simulink model "exampleModel_bus_axi_w_4ptavg"  (R2017b)
settings: Solver=VariableStepAuto  StartTime=0.0  StopTime=10e-5  RelTol=1e-3
PreLoadFcn:
  | setup
values from neighbouring files (symbols this model uses):
  axiClk = 156.25e6    (= 156250000)    [setup.m]    (also in setup_exampleModel_bus_axi_simulink.m; setup_exampleModel_bus_axi_simulink_lcls2.m; setup_lcls2_pcav.m; sysgen_signal.m)
  cav1p1_addr = 204    [setup_exampleModel_bus_axi_simulink.m]    (also in setup_exampleModel_bus_axi_simulink_lcls2.m; setup_lcls2_pcav.m; sysgen_signal.m)
  cav1p2_addr = cav1p1_addr * 2    (= 408)    [setup_exampleModel_bus_axi_simulink.m]    (also in setup_exampleModel_bus_axi_simulink_lcls2.m; setup_lcls2_pcav.m; sysgen_signal.m)
  cav2p1_addr = cav1p1_addr * 3    (= 612)    [setup_exampleModel_bus_axi_simulink.m]    (also in setup_exampleModel_bus_axi_simulink_lcls2.m; setup_lcls2_pcav.m; sysgen_signal.m)
  cav2p2_addr = cav1p1_addr * 4    (= 816)    [setup_exampleModel_bus_axi_simulink.m]    (also in setup_exampleModel_bus_axi_simulink_lcls2.m; setup_lcls2_pcav.m; sysgen_signal.m)
  Fadc = Fs/interleavedChannels    (= 29750000)    [setup.m]    (also in setup_exampleModel_bus_axi_simulink.m = 357000000; setup_exampleModel_bus_axi_simulink_lcls2.m = 351000000; setup_lcls2_pcav.m = 357000000; sysgen_signal.m = 357000000)
  fir_lpf = fir1(15, w_lpf)    [setup_exampleModel_bus_axi_simulink.m]    (also in setup_exampleModel_bus_axi_simulink_lcls2.m; setup_lcls2_pcav.m)
  Fproc = 204e6    (= 204000000)    [setup_exampleModel_bus_axi_simulink.m]    (also in setup_exampleModel_bus_axi_simulink_lcls2.m = 200571400; setup_lcls2_pcav.m; sysgen_signal.m)
  Fsig = Fproc/12    (= 17000000)    [setup_exampleModel_bus_axi_simulink.m]    (also in setup_exampleModel_bus_axi_simulink_lcls2.m = 16714283.3333; setup_lcls2_pcav.m)
  Tadc = 1/fadc    (= 2.80112044818e-09)    [cavity_signal.m]    (also in setup_exampleModel_bus_axi_simulink.m; setup_exampleModel_bus_axi_simulink_lcls2.m = 2.849002849e-09; setup_lcls2_pcav.m; setup_pcav_simulink.m)
undefined symbols (not defined in the file or in its folder): AXI4, Lite
libraries: xbsIndex_r4 x2870, llrf_lib x10, simulink x3
(part 7 of 15)

== system exampleModel_bus_axi_w_4ptavg/example/dsp/Cav1/Subsystem ==
  In1 : Inport
  In2 : Inport  Port=2
  In3 : Inport  Port=3
  In4 : Inport  Port=4
  AddSub1 : xbsIndex_r4/AddSub  mode=Addition  use_carryin=off  use_carryout=off  en=off  latency=1  precision=User Defined  arith_type=Unsigned  n_bits=16  bin_pt=0  quantization=Truncate  overflow=Wrap  use_behavioral_HDL=off  hw_selection=Fabric  pipelined=off  dbl_ovrd=off  block_type=addsub
  AddSub2 : xbsIndex_r4/AddSub  mode=Addition  use_carryin=off  use_carryout=off  en=off  latency=1  precision=User Defined  arith_type=Unsigned  n_bits=16  bin_pt=0  quantization=Truncate  overflow=Wrap  use_behavioral_HDL=off  hw_selection=Fabric  pipelined=off  dbl_ovrd=off  block_type=addsub
  CORDIC 6.0 1 : xbsIndex_r4/CORDIC 6.0   functional_selection=Translate  architectural_configuration=Parallel  pipelining_mode=Maximum  data_format=SignedFraction  phase_format=Scaled_Radians  input_width=33  output_width=33  round_mode=Truncate  iterations=0  precision=0  compensation_scaling=No_Scale_Compensation  coarse_rotation=on  aclken=off  aresetn=off  out_tready=off  cartesian_has_tuser=off  cartesian_has_tlast=off  cartesian_tuser_width=1  phase_has_tuser=off  phase_has_tlast=off  phase_tuser_width=1  out_tlast_behv=Null  flow_control=NonBlocking  optimize_goal=Resources  trim_axipin_name=on  simulation_type=hybrid_sim  simulation_model=sysgen:cordic_v6_0  data_path_portlist={'s_axis_cartesian_tdata_imag', 's_axis_cartesian_tdata_real', 's_axis_phase_tdata_phase', 'm_axis_dout_tdata_imag', 'm_axis_dout_tdata_real', 'm_axis_dout_tdata_phase','m_axis_dout_tdata'}  ip_name=CORDIC  ip_version=6.0  dsptool_ready=true  ipcore_usecache=true  ipcore_useipmodelcache=true  wrapper_available=true  port_translation_map={ 'aclken' => 'en', 'aresetn' => 'rst' }  block_type=cordic_v6_0
      settings: infoedit=CORDIC 6.0
  Clock Enable Probe3 : xbsIndex_r4/Clock Enable Probe  inherit_constraints=on  block_type=ceprobe
      settings: infoedit="Clock enable extractor.  Produces a Boolean output that mirrors the hardware clock enable associated with the input sample rate.<br><br>Hardware notes: in hardware this block costs nothing."
  Constant13 : xbsIndex_r4/Constant  const=0  gui_display_data_type=Boolean  arith_type=Boolean  n_bits=16  bin_pt=14  preci_type=Single  exp_width=8  frac_width=24  explicit_period=off  period=1  equ=P=C  opselect=C  inp2=PCIN>>17  opr=+  inp1=P  carry=CIN  dbl_ovrd=off  block_type=constant
  Constant15 : xbsIndex_r4/Constant  const=0  gui_display_data_type=Fixed-point  arith_type=Signed (2's comp)  n_bits=33  bin_pt=31  preci_type=Single  exp_width=8  frac_width=24  explicit_period=off  period=1  equ=P=C  opselect=C  inp2=PCIN>>17  opr=+  inp1=P  carry=CIN  dbl_ovrd=off  block_type=constant
  Constant3 : xbsIndex_r4/Constant  const=1.0  gui_display_data_type=Boolean  arith_type=Boolean  n_bits=16  bin_pt=14  preci_type=Single  exp_width=8  frac_width=24  explicit_period=off  period=1  equ=P=C  opselect=C  inp2=PCIN>>17  opr=+  inp1=P  carry=CIN  dbl_ovrd=off  block_type=constant
  Constant4 : xbsIndex_r4/Constant  const=0  gui_display_data_type=Boolean  arith_type=Boolean  n_bits=16  bin_pt=14  preci_type=Single  exp_width=8  frac_width=24  explicit_period=off  period=1  equ=P=C  opselect=C  inp2=PCIN>>17  opr=+  inp1=P  carry=CIN  dbl_ovrd=off  block_type=constant
  Constant5 : xbsIndex_r4/Constant  const=0  gui_display_data_type=Fixed-point  arith_type=Signed (2's comp)  n_bits=33  bin_pt=31  preci_type=Single  exp_width=8  frac_width=24  explicit_period=off  period=1  equ=P=C  opselect=C  inp2=PCIN>>17  opr=+  inp1=P  carry=CIN  dbl_ovrd=off  block_type=constant
  Constant6 : xbsIndex_r4/Constant  const=1.0  gui_display_data_type=Boolean  arith_type=Boolean  n_bits=16  bin_pt=14  preci_type=Single  exp_width=8  frac_width=24  explicit_period=off  period=1  equ=P=C  opselect=C  inp2=PCIN>>17  opr=+  inp1=P  carry=CIN  dbl_ovrd=off  block_type=constant
  Down Sample8 : xbsIndex_r4/Down Sample  sample_ratio=12  sample_phase="Last Value of Frame  (most efficient)"  en=off  rst=off  latency=1  dbl_ovrd=off  block_type=dsamp
  Dual Port RAM : xbsIndex_r4/Dual Port RAM  depth=2^16  initVector=zeros(1,2^8)  distributed_mem=Block RAM  init_a=0  init_b=0  rst_a=off  rst_b=off  en_a=off  en_b=off  latency=1  write_mode_A=Read Before Write  write_mode_B=Read Before Write  optimize=Area  dbl_ovrd=off  block_type=dpram
  Dual Port RAM1 : xbsIndex_r4/Dual Port RAM  depth=2^16  initVector=zeros(1,2^8)  distributed_mem=Block RAM  init_a=0  init_b=0  rst_a=off  rst_b=off  en_a=off  en_b=off  latency=1  write_mode_A=Read Before Write  write_mode_B=Read Before Write  optimize=Area  dbl_ovrd=off  block_type=dpram
  Gateway Out{7..11,20,22..24} (9 alike) : xbsIndex_r4/Gateway Out  inherit_from_input=off  hdl_port=off  rows=1  columns=1  UseAsDAC=off  DACChannel='1'  interface=None  automatic_assignment=on  address_offset=hex2dec('00')  intf_name=''  intf_description=''  timing_constraint=None  locs_specified=off  LOCs={}  io_standard={}  block_type=gatewayout
  Gateway Out{12..13,15,21,29} (5 alike) : xbsIndex_r4/Gateway Out  inherit_from_input=off  hdl_port=on  rows=1  columns=1  UseAsDAC=off  DACChannel='1'  interface=None  automatic_assignment=on  address_offset=hex2dec('00')  intf_name=''  intf_description=''  timing_constraint=None  locs_specified=off  LOCs={}  io_standard={}  block_type=gatewayout
  Mult1 : xbsIndex_r4/Mult  precision=User Defined  arith_type="Signed  (2's comp)"  n_bits=33  bin_pt=31  quantization=Truncate  overflow=Wrap  en=off  latency=3  use_behavioral_HDL=off  opt=Speed  use_embedded=on  optimum_pipeline=off  pipeline=on  dbl_ovrd=off  use_rpm=on  placement_style=Triangular  block_type=mult
  Mult3 : xbsIndex_r4/Mult  precision=User Defined  arith_type="Signed  (2's comp)"  n_bits=33  bin_pt=31  quantization=Truncate  overflow=Saturate  en=off  latency=3  use_behavioral_HDL=off  opt=Speed  use_embedded=on  optimum_pipeline=off  pipeline=on  dbl_ovrd=off  use_rpm=on  placement_style=Triangular  block_type=mult
  Scope10 : Scope  NumInputPorts=2
  Scope3 : Scope  NumInputPorts=3
  Scope6 : Scope  NumInputPorts=3
  Scope7 : Scope  NumInputPorts=4
  Scope8 : Scope  NumInputPorts=4
  Scope9 : Scope  NumInputPorts=2
  four_point_avg : Subsystem
  freq_err : Subsystem
  Out1 : Outport
  tag scope: Cav1_NCO_fb=global, delayed_test_img=global, delayed_test_real=global
  wires:
  In4/1 -> Scope7/4
  In3/1 -> Scope8/4
  In1/1 -> Scope3/3
  freq_err/1(NCO_err) -> [Cav1_NCO_fb]
  Gateway Out15/1 -> Scope7/2
  Dual Port RAM1/2 -> Gateway Out24/1, [delayed_test_real]
  Gateway Out24/1 -> Scope10/2
  [c1p2_pt_cntr] -> AddSub1/2, Dual Port RAM/4
  Constant15/1 -> Dual Port RAM/5
  Dual Port RAM/1 -> Gateway Out20/1
  [c1p2_pt_cntr] -> Dual Port RAM1/4, AddSub2/2
  AddSub2/1 -> Dual Port RAM1/1
  Gateway Out13/1 -> Scope8/3
  Constant13/1 -> Dual Port RAM/6
  Constant6/1 -> Dual Port RAM1/3
  In2/1 -> Scope7/3
  [c1p2_window_func] -> Mult3/2
  [test_img] -> Dual Port RAM/2
  Gateway Out22/1 -> Scope9/2
  AddSub1/1 -> Dual Port RAM/1
  Dual Port RAM1/1 -> Gateway Out23/1
  Constant5/1 -> Dual Port RAM1/5
  Gateway Out20/1 -> Scope9/1
  Constant3/1 -> Dual Port RAM/3
  CORDIC 6.0 1/3 -> Gateway Out9/1, Gateway Out7/1, four_point_avg/1(In1)
  CORDIC 6.0 1/1 -> Out1/1
  Gateway Out9/1 -> Scope6/1
  Clock Enable Probe3/1 -> Down Sample8/1
  Gateway Out23/1 -> Scope10/1
  [c1p2_delay_match] -> AddSub2/1
  Gateway Out11/1 -> Scope6/3
  Gateway Out21/1 -> Scope7/1
  Mult1/1 -> Gateway Out15/1, CORDIC 6.0 1/3
  Mult3/1 -> Gateway Out21/1, Clock Enable Probe3/1, CORDIC 6.0 1/2
  [c1p2_pt_cntr] -> Gateway Out11/1
  [delayed_test_img] -> Gateway Out29/1, Mult3/1
  Gateway Out12/1 -> Scope8/2
  Down Sample8/1 -> CORDIC 6.0 1/1
  [flo_c1p2_window] -> freq_err/2(window)
  [test_real] -> Dual Port RAM1/2
  Constant4/1 -> Dual Port RAM1/6
  [c1p2_window_func] -> Gateway Out13/1, Mult1/2
  Dual Port RAM/2 -> [delayed_test_img], Gateway Out22/1
  Gateway Out8/1 -> Scope3/2
  [dsp_cav1_reset] -> freq_err/3(reset)
  [delayed_test_real] -> Gateway Out12/1, Mult1/1
  CORDIC 6.0 1/2 -> Gateway Out10/1, freq_err/1(raw_phase)
  four_point_avg/1(Out1) -> Gateway Out8/1
  Gateway Out7/1 -> Scope3/1
  Gateway Out10/1 -> Scope6/2
  Gateway Out29/1 -> Scope8/1
  [c1p2_delay_match] -> AddSub1/1

== system exampleModel_bus_axi_w_4ptavg/example/dsp/Cav1/Subsystem1 ==
  IQ_stream_in : Inport
  IQ_chan_sel : Inport  Port=2
  Bus Creator5 : BusCreator  Inputs=3
  Bus Selector : BusSelector  OutputSignals=ddcI,ddcQ,sync
  Bus Selector3 : BusSelector  OutputSignals=ddcI,ddcQ,ddcSync,ddcChannel
  Channel Select3 : llrf_lib/Sysgen/Single Rate/Channel Select  SystemSampleTime=-1
      settings: SourceProductName=LLRF Library
  ddcI : Outport
  ddcQ : Outport  Port=2
  sync : Outport  Port=3
  wires:
  IQ_stream_in/1 -> Bus Selector3/1
  IQ_chan_sel/1 -> Channel Select3/5
  Channel Select3/3 -> Bus Creator5/3  "sync"
  Bus Selector3/2 -> Channel Select3/2  "<ddcQ>"
  Channel Select3/1 -> Bus Creator5/1  "ddcI"
  Channel Select3/2 -> Bus Creator5/2  "ddcQ"
  Bus Selector3/1 -> Channel Select3/1  "<ddcI>"
  Bus Selector3/4 -> Channel Select3/4  "<ddcChannel>"
  Bus Selector3/3 -> Channel Select3/3  "<ddcSync>"
  Bus Creator5/1 -> Bus Selector/1
  Bus Selector/1 -> ddcI/1  "<ddcI>"
  Bus Selector/2 -> ddcQ/1  "<ddcQ>"
  Bus Selector/3 -> sync/1  "<sync>"

== system exampleModel_bus_axi_w_4ptavg/example/dsp/Cav1/Subsystem10 ==
  d : Inport
  reset : Inport  Port=2
  cntr : Inport  Port=3
  threshold : Inport  Port=4
  Register11 : xbsIndex_r4/Register  init=0  rst=on  en=on  dbl_ovrd=off  block_type=register
  Relational4 : xbsIndex_r4/Relational  mode=a>b  op_type=Bool  en=off  latency=1  dbl_ovrd=off  block_type=relational
  posedge_pulse : Subsystem
  q : Outport
  wires:
  threshold/1 -> Relational4/2
  reset/1 -> Register11/2
  Relational4/1 -> posedge_pulse/1(In1)
  posedge_pulse/1(Out1) -> Register11/3
  Register11/1 -> q/1
  cntr/1 -> Relational4/1
  d/1 -> Register11/1

== system exampleModel_bus_axi_w_4ptavg/example/dsp/Cav1/Subsystem11 ==
  d : Inport
  reset : Inport  Port=2
  cntr : Inport  Port=3
  threshold : Inport  Port=4
  Register11 : xbsIndex_r4/Register  init=0  rst=on  en=on  dbl_ovrd=off  block_type=register
  Relational4 : xbsIndex_r4/Relational  mode=a>b  op_type=Bool  en=off  latency=1  dbl_ovrd=off  block_type=relational
  posedge_pulse : Subsystem
  q : Outport
  wires:
  d/1 -> Register11/1
  cntr/1 -> Relational4/1
  Register11/1 -> q/1
  posedge_pulse/1(Out1) -> Register11/3
  Relational4/1 -> posedge_pulse/1(In1)
  reset/1 -> Register11/2
  threshold/1 -> Relational4/2

== system exampleModel_bus_axi_w_4ptavg/example/dsp/Cav1/Subsystem12 ==
  d : Inport
  reset : Inport  Port=2
  cntr : Inport  Port=3
  threshold : Inport  Port=4
  Register11 : xbsIndex_r4/Register  init=0  rst=on  en=on  dbl_ovrd=off  block_type=register
  Relational4 : xbsIndex_r4/Relational  mode=a>b  op_type=Bool  en=off  latency=1  dbl_ovrd=off  block_type=relational
  posedge_pulse : Subsystem
  q : Outport
  wires:
  threshold/1 -> Relational4/2
  reset/1 -> Register11/2
  Relational4/1 -> posedge_pulse/1(In1)
  posedge_pulse/1(Out1) -> Register11/3
  Register11/1 -> q/1
  cntr/1 -> Relational4/1
  d/1 -> Register11/1

== system exampleModel_bus_axi_w_4ptavg/example/dsp/Cav1/Subsystem13 ==
  d : Inport
  reset : Inport  Port=2
  cntr : Inport  Port=3
  threshold : Inport  Port=4
  Register11 : xbsIndex_r4/Register  init=0  rst=on  en=on  dbl_ovrd=off  block_type=register
  Relational4 : xbsIndex_r4/Relational  mode=a>b  op_type=Bool  en=off  latency=1  dbl_ovrd=off  block_type=relational
  posedge_pulse : Subsystem
  q : Outport
  wires:
  d/1 -> Register11/1
  cntr/1 -> Relational4/1
  Register11/1 -> q/1
  posedge_pulse/1(Out1) -> Register11/3
  Relational4/1 -> posedge_pulse/1(In1)
  reset/1 -> Register11/2
  threshold/1 -> Relational4/2

== system exampleModel_bus_axi_w_4ptavg/example/dsp/Cav1/Subsystem2 ==
  In1 : Inport
  Delay4 : xbsIndex_r4/Delay  rst=off  infoeditControl=Selection of Reset will increase slice count due to use of real FFs and instead of SRLs  en=off  latency=15  reg_retiming=off  dbl_ovrd=off  block_type=delay
  Inverter : xbsIndex_r4/Inverter  en=off  latency=20  dbl_ovrd=off  block_type=inv
  Inverter8 : xbsIndex_r4/Inverter  en=off  latency=1  dbl_ovrd=off  block_type=inv
  Logical : xbsIndex_r4/Logical  logical_function=AND  inputs=2  en=off  latency=1  precision=User Defined  arith_type=Boolean  n_bits=1  bin_pt=0  align_bp=on  dbl_ovrd=off  block_type=logical
  Out1 : Outport
  wires:
  Logical/1 -> Delay4/1
  In1/1 -> Inverter8/1
  Delay4/1 -> Out1/1
  Inverter/1 -> Logical/2
  Inverter8/1 -> Logical/1, Inverter/1

== system exampleModel_bus_axi_w_4ptavg/example/dsp/Cav1/Subsystem3 ==
  IQ_stream_in : Inport
  IQ_chan_sel : Inport  Port=2
  Bus Creator5 : BusCreator  Inputs=3
  Bus Selector : BusSelector  OutputSignals=ddcI,ddcQ,sync
  Bus Selector3 : BusSelector  OutputSignals=ddcI,ddcQ,ddcSync,ddcChannel
  Channel Select3 : llrf_lib/Sysgen/Single Rate/Channel Select  SystemSampleTime=-1
      settings: SourceProductName=LLRF Library
  ddcI : Outport
  ddcQ : Outport  Port=2
  sync : Outport  Port=3
  wires:
  Bus Selector/3 -> sync/1  "<sync>"
  Bus Selector/2 -> ddcQ/1  "<ddcQ>"
  Bus Selector/1 -> ddcI/1  "<ddcI>"
  Bus Creator5/1 -> Bus Selector/1
  Bus Selector3/3 -> Channel Select3/3  "<ddcSync>"
  Bus Selector3/4 -> Channel Select3/4  "<ddcChannel>"
  Bus Selector3/1 -> Channel Select3/1  "<ddcI>"
  Channel Select3/2 -> Bus Creator5/2  "ddcQ"
  Channel Select3/1 -> Bus Creator5/1  "ddcI"
  Bus Selector3/2 -> Channel Select3/2  "<ddcQ>"
  Channel Select3/3 -> Bus Creator5/3  "sync"
  IQ_chan_sel/1 -> Channel Select3/5
  IQ_stream_in/1 -> Bus Selector3/1

== system exampleModel_bus_axi_w_4ptavg/example/dsp/Cav1/Subsystem4 ==
  d : Inport
  reset : Inport  Port=2
  cntr : Inport  Port=3
  threshold : Inport  Port=4
  Gateway Out{1,7..9} (4 alike) : xbsIndex_r4/Gateway Out  inherit_from_input=off  hdl_port=on  rows=1  columns=1  UseAsDAC=off  DACChannel='1'  interface=None  automatic_assignment=on  address_offset=hex2dec('00')  intf_name=''  intf_description=''  timing_constraint=None  locs_specified=off  LOCs={}  io_standard={}  block_type=gatewayout
  Register11 : xbsIndex_r4/Register  init=0  rst=on  en=on  dbl_ovrd=off  block_type=register
  Relational4 : xbsIndex_r4/Relational  mode=a>b  op_type=Bool  en=off  latency=1  dbl_ovrd=off  block_type=relational
  Scope3 : Scope  NumInputPorts=4
  posedge_pulse : Subsystem
  q : Outport
  wires:
  d/1 -> Gateway Out7/1, Register11/1
  cntr/1 -> Relational4/1
  Register11/1 -> Gateway Out8/1, q/1
  posedge_pulse/1(Out1) -> Register11/3, Gateway Out1/1
  Relational4/1 -> posedge_pulse/1(In1)
  reset/1 -> Gateway Out9/1, Register11/2
  threshold/1 -> Relational4/2
  Gateway Out1/1 -> Scope3/4
  Gateway Out7/1 -> Scope3/1
  Gateway Out8/1 -> Scope3/2
  Gateway Out9/1 -> Scope3/3

== system exampleModel_bus_axi_w_4ptavg/example/dsp/Cav1/Subsystem5 ==
  d : Inport
  reset : Inport  Port=2
  cntr : Inport  Port=3
  threshold : Inport  Port=4
  Register11 : xbsIndex_r4/Register  init=0  rst=on  en=on  dbl_ovrd=off  block_type=register
  Relational4 : xbsIndex_r4/Relational  mode=a>b  op_type=Bool  en=off  latency=1  dbl_ovrd=off  block_type=relational
  posedge_pulse : Subsystem
  q : Outport
  wires:
  threshold/1 -> Relational4/2
  reset/1 -> Register11/2
  Relational4/1 -> posedge_pulse/1(In1)
  posedge_pulse/1(Out1) -> Register11/3
  Register11/1 -> q/1
  cntr/1 -> Relational4/1
  d/1 -> Register11/1

== system exampleModel_bus_axi_w_4ptavg/example/dsp/Cav1/Subsystem6 ==
  d : Inport
  reset : Inport  Port=2
  cntr : Inport  Port=3
  threshold : Inport  Port=4
  Register11 : xbsIndex_r4/Register  init=0  rst=on  en=on  dbl_ovrd=off  block_type=register
  Relational4 : xbsIndex_r4/Relational  mode=a>b  op_type=Bool  en=off  latency=1  dbl_ovrd=off  block_type=relational
  posedge_pulse : Subsystem
  q : Outport
  wires:
  threshold/1 -> Relational4/2
  reset/1 -> Register11/2
  Relational4/1 -> posedge_pulse/1(In1)
  posedge_pulse/1(Out1) -> Register11/3
  Register11/1 -> q/1
  cntr/1 -> Relational4/1
  d/1 -> Register11/1

== system exampleModel_bus_axi_w_4ptavg/example/dsp/Cav1/Subsystem7 ==
  d : Inport
  reset : Inport  Port=2
  cntr : Inport  Port=3
  threshold : Inport  Port=4
  Register11 : xbsIndex_r4/Register  init=0  rst=on  en=on  dbl_ovrd=off  block_type=register
  Relational4 : xbsIndex_r4/Relational  mode=a>b  op_type=Bool  en=off  latency=1  dbl_ovrd=off  block_type=relational
  posedge_pulse : Subsystem
  q : Outport
  wires:
  d/1 -> Register11/1
  cntr/1 -> Relational4/1
  Register11/1 -> q/1
  posedge_pulse/1(Out1) -> Register11/3
  Relational4/1 -> posedge_pulse/1(In1)
  reset/1 -> Register11/2
  threshold/1 -> Relational4/2

== system exampleModel_bus_axi_w_4ptavg/example/dsp/Cav1/Subsystem8 ==
  d : Inport
  reset : Inport  Port=2
  cntr : Inport  Port=3
  threshold : Inport  Port=4
  Register11 : xbsIndex_r4/Register  init=0  rst=on  en=on  dbl_ovrd=off  block_type=register
  Relational4 : xbsIndex_r4/Relational  mode=a>b  op_type=Bool  en=off  latency=1  dbl_ovrd=off  block_type=relational
  posedge_pulse : Subsystem
  q : Outport
  wires:
  threshold/1 -> Relational4/2
  reset/1 -> Register11/2
  Relational4/1 -> posedge_pulse/1(In1)
  posedge_pulse/1(Out1) -> Register11/3
  Register11/1 -> q/1
  cntr/1 -> Relational4/1
  d/1 -> Register11/1

== system exampleModel_bus_axi_w_4ptavg/example/dsp/Cav1/Subsystem9 ==
  d : Inport
  reset : Inport  Port=2
  cntr : Inport  Port=3
  threshold : Inport  Port=4
  Register11 : xbsIndex_r4/Register  init=0  rst=on  en=on  dbl_ovrd=off  block_type=register
  Relational4 : xbsIndex_r4/Relational  mode=a>b  op_type=Bool  en=off  latency=1  dbl_ovrd=off  block_type=relational
  posedge_pulse : Subsystem
  q : Outport
  wires:
  d/1 -> Register11/1
  cntr/1 -> Relational4/1
  Register11/1 -> q/1
  posedge_pulse/1(Out1) -> Register11/3
  Relational4/1 -> posedge_pulse/1(In1)
  reset/1 -> Register11/2
  threshold/1 -> Relational4/2

== system exampleModel_bus_axi_w_4ptavg/example/dsp/Cav1/c1p1_Masking_window ==
  note: delay for the comparison because Axilite register
      | takes a about 40 dsp clk cycles to load in
  phi_reset_trig : Inport
  start_pt : Inport  Port=2
  stop_pt : Inport  Port=3
  delay_amt : Inport  Port=4
  delay_latch : Inport  Port=5
  AddSub1 : xbsIndex_r4/AddSub  mode=Addition  use_carryin=off  use_carryout=off  en=off  latency=1  precision=User Defined  arith_type=Unsigned  n_bits=16  bin_pt=0  quantization=Truncate  overflow=Wrap  use_behavioral_HDL=off  hw_selection=Fabric  pipelined=off  dbl_ovrd=off  block_type=addsub
  AddSub4 : xbsIndex_r4/AddSub  mode=Addition  use_carryin=off  use_carryout=off  en=on  latency=1  precision=User Defined  arith_type=Unsigned  n_bits=16  bin_pt=0  quantization=Truncate  overflow=Saturate  use_behavioral_HDL=off  hw_selection=Fabric  pipelined=off  dbl_ovrd=off  block_type=addsub
  Constant1 : xbsIndex_r4/Constant  const=40  gui_display_data_type=Fixed-point  arith_type=Unsigned  n_bits=16  bin_pt=0  preci_type=Single  exp_width=8  frac_width=24  explicit_period=off  period=1  equ=P=C  opselect=C  inp2=PCIN>>17  opr=+  inp1=P  carry=CIN  dbl_ovrd=off  block_type=constant
  Constant11 : xbsIndex_r4/Constant  const=55  gui_display_data_type=Fixed-point  arith_type=Unsigned  n_bits=16  bin_pt=0  preci_type=Single  exp_width=8  frac_width=24  explicit_period=off  period=1  equ=P=C  opselect=C  inp2=PCIN>>17  opr=+  inp1=P  carry=CIN  dbl_ovrd=off  block_type=constant
  Constant2 : xbsIndex_r4/Constant  const=106  gui_display_data_type=Fixed-point  arith_type=Unsigned  n_bits=16  bin_pt=0  preci_type=Single  exp_width=8  frac_width=24  explicit_period=off  period=1  equ=P=C  opselect=C  inp2=PCIN>>17  opr=+  inp1=P  carry=CIN  dbl_ovrd=off  block_type=constant
  Constant3 : xbsIndex_r4/Constant  const=88  gui_display_data_type=Fixed-point  arith_type=Unsigned  n_bits=16  bin_pt=0  preci_type=Single  exp_width=8  frac_width=24  explicit_period=off  period=1  equ=P=C  opselect=C  inp2=PCIN>>17  opr=+  inp1=P  carry=CIN  dbl_ovrd=off  block_type=constant
  Convert{1,4..5,7..8} (5 alike) : xbsIndex_r4/Convert  gui_display_data_type=Boolean  arith_type=Boolean  n_bits=1  bin_pt=0  float_type=Single  exp_bits=8  fraction_bits=24  quantization=Truncate  overflow=Wrap  en=off  latency=1  pipeline=off  dbl_ovrd=off  block_type=convert
  Convert11 : xbsIndex_r4/Convert  gui_display_data_type=Fixed-point  arith_type=Unsigned  n_bits=1  bin_pt=0  float_type=Single  exp_bits=8  fraction_bits=24  quantization=Truncate  overflow=Wrap  en=off  latency=1  pipeline=off  dbl_ovrd=off  block_type=convert
  Convert2 : xbsIndex_r4/Convert  gui_display_data_type=Fixed-point  arith_type=Unsigned  n_bits=1  bin_pt=0  float_type=Single  exp_bits=8  fraction_bits=24  quantization=Truncate  overflow=Wrap  en=off  latency=1  pipeline=off  dbl_ovrd=off  block_type=convert
  Convert3 : xbsIndex_r4/Convert  gui_display_data_type=Boolean  arith_type=Boolean  n_bits=16  bin_pt=14  float_type=Single  exp_bits=8  fraction_bits=24  quantization=Truncate  overflow=Wrap  en=off  latency=1  pipeline=off  dbl_ovrd=off  block_type=convert
  Convert6 : xbsIndex_r4/Convert  gui_display_data_type=Fixed-point  arith_type=Unsigned  n_bits=8  bin_pt=0  float_type=Single  exp_bits=8  fraction_bits=24  quantization=Truncate  overflow=Saturate  en=off  latency=1  pipeline=off  dbl_ovrd=off  block_type=convert
  Counter : xbsIndex_r4/Counter  cnt_type=Count Limited  cnt_to=(2^15)  operation=Up  start_count=0  cnt_by_val=1  arith_type=Unsigned  n_bits=16  bin_pt=0  load_pin=off  rst=on  en=on  explicit_period=on  period=12/Fproc  use_behavioral_HDL=off  implementation=Fabric  dbl_ovrd=off  block_type=counter
  Delay{,1..4,6..7} (7 alike) : xbsIndex_r4/Delay  rst=off  infoeditControl=Selection of Reset will increase slice count due to use of real FFs and instead of SRLs  en=off  latency=1  reg_retiming=off  dbl_ovrd=off  block_type=delay
  Delay5 : xbsIndex_r4/Delay  rst=off  infoeditControl=Selection of Reset will increase slice count due to use of real FFs and instead of SRLs  en=off  latency=3  reg_retiming=off  dbl_ovrd=off  block_type=delay
  Display1 : Display
  Down Sample1 : xbsIndex_r4/Down Sample  sample_ratio=12  sample_phase="Last Value of Frame  (most efficient)"  en=off  rst=off  latency=1  dbl_ovrd=off  block_type=dsamp
  Down Sample2 : xbsIndex_r4/Down Sample  sample_ratio=12  sample_phase="Last Value of Frame  (most efficient)"  en=off  rst=off  latency=1  dbl_ovrd=off  block_type=dsamp
  Gateway Out{1..3,5,27..29} (7 alike) : xbsIndex_r4/Gateway Out  inherit_from_input=off  hdl_port=on  rows=1  columns=1  UseAsDAC=off  DACChannel='1'  interface=None  automatic_assignment=on  address_offset=hex2dec('00')  intf_name=''  intf_description=''  timing_constraint=None  locs_specified=off  LOCs={}  io_standard={}  block_type=gatewayout
  Gateway Out16 : xbsIndex_r4/Gateway Out  inherit_from_input=off  hdl_port=off  rows=1  columns=1  UseAsDAC=off  DACChannel='1'  interface=None  automatic_assignment=on  address_offset=hex2dec('00')  intf_name=''  intf_description=''  timing_constraint=None  locs_specified=off  LOCs={}  io_standard={}  block_type=gatewayout
  Gateway Out17 : xbsIndex_r4/Gateway Out  inherit_from_input=off  hdl_port=off  rows=1  columns=1  UseAsDAC=off  DACChannel='1'  interface=None  automatic_assignment=on  address_offset=hex2dec('00')  intf_name=''  intf_description=''  timing_constraint=None  locs_specified=off  LOCs={}  io_standard={}  block_type=gatewayout
  Gateway Out18 : xbsIndex_r4/Gateway Out  inherit_from_input=off  hdl_port=off  rows=1  columns=1  UseAsDAC=off  DACChannel='1'  interface=None  automatic_assignment=on  address_offset=hex2dec('00')  intf_name=''  intf_description=''  timing_constraint=None  locs_specified=off  LOCs={}  io_standard={}  block_type=gatewayout
  Logical1 : xbsIndex_r4/Logical  logical_function=AND  inputs=2  en=off  latency=1  precision=Full  arith_type=Unsigned  n_bits=16  bin_pt=0  align_bp=on  dbl_ovrd=off  block_type=logical
  Logical2 : xbsIndex_r4/Logical  logical_function=AND  inputs=2  en=off  latency=1  precision=Full  arith_type=Unsigned  n_bits=16  bin_pt=0  align_bp=on  dbl_ovrd=off  block_type=logical
  Register : xbsIndex_r4/Register  init=44  rst=off  en=on  dbl_ovrd=off  block_type=register
  Register1 : xbsIndex_r4/Register  init=0  rst=off  en=on  dbl_ovrd=off  block_type=register
  Register10 : xbsIndex_r4/Register  init=0  rst=off  en=off  dbl_ovrd=off  block_type=register
  Register5 : xbsIndex_r4/Register  init=0  rst=off  en=off  dbl_ovrd=off  block_type=register
  Register6 : xbsIndex_r4/Register  init=100  rst=off  en=off  dbl_ovrd=off  block_type=register
  Relational1 : xbsIndex_r4/Relational  mode=a<b  op_type=Bool  en=on  latency=1  dbl_ovrd=off  block_type=relational
  Relational2 : xbsIndex_r4/Relational  mode=a>b  op_type=Bool  en=off  latency=1  dbl_ovrd=off  block_type=relational
  Relational3 : xbsIndex_r4/Relational  mode=a<b  op_type=Bool  en=on  latency=1  dbl_ovrd=off  block_type=relational
  Relational4 : xbsIndex_r4/Relational  mode=a>b  op_type=Bool  en=on  latency=1  dbl_ovrd=off  block_type=relational
  Relational5 : xbsIndex_r4/Relational  mode=a<b  op_type=Bool  en=on  latency=1  dbl_ovrd=off  block_type=relational
  Relational6 : xbsIndex_r4/Relational  mode=a>=b  op_type=Bool  en=on  latency=1  dbl_ovrd=off  block_type=relational
  Scope1 : Scope  NumInputPorts=3
  Scope10 : Scope  NumInputPorts=3
  Scope2 : Scope  NumInputPorts=2
  Scope5 : Scope  NumInputPorts=3
  counter : Outport
  eval_window : Outport  Port=2
  integral_trig : Outport  Port=3
  flo_window : Outport  Port=4
  delay_val : Outport  Port=5
  wires:
  Gateway Out5/1 -> Scope2/2
  start_pt/1 -> Register5/1
  phi_reset_trig/1 -> Register10/1
  Register5/1 -> Down Sample1/1
  stop_pt/1 -> Register6/1
  Register6/1 -> Down Sample2/1
  Delay2/1 -> Relational4/2
  Delay3/1 -> AddSub1/1, Gateway Out2/1, Relational3/2
  Constant1/1 -> Relational2/2
  Relational3/1 -> Gateway Out28/1, Convert7/1
  Relational4/1 -> Gateway Out27/1, Convert8/1
  Gateway Out28/1 -> Scope10/2
  Gateway Out29/1 -> Scope2/1, Scope10/3
  Gateway Out27/1 -> Scope10/1
  Logical1/1 -> Convert11/1
  Convert8/1 -> Logical1/1
  Convert7/1 -> Gateway Out3/1, Logical1/2
  Convert11/1 -> eval_window/1, Gateway Out29/1
  Convert5/1 -> integral_trig/1, Gateway Out5/1
  Relational5/1 -> Convert5/1
  Relational2/1 -> Relational6/3, Relational1/3, Relational5/3, Relational3/3, Relational4/3
  Counter/1 -> Convert6/1
  Constant11/1 -> AddSub1/2
  AddSub1/1 -> Relational5/2
  Register10/1 -> Convert3/1
  Down Sample1/1 -> Delay2/1
  Down Sample2/1 -> Delay3/1
  Gateway Out1/1 -> Scope1/1
  Gateway Out2/1 -> Scope1/2
  Gateway Out3/1 -> Scope1/3
  Delay1/1 -> Relational4/1
  Delay4/1 -> Relational3/1
  Delay5/1 -> Gateway Out1/1
  Delay7/1 -> Relational1/1
  Constant2/1 -> Relational1/2
  Relational1/1 -> Convert1/1
  Logical2/1 -> Convert2/1
  Convert1/1 -> Logical2/2
  Convert2/1 -> flo_window/1
  Delay6/1 -> Relational6/1
  Constant3/1 -> Relational6/2
  Relational6/1 -> Convert4/1
  Convert4/1 -> Logical2/1
  Gateway Out18/1 -> Scope5/3
  delay_latch/1 -> Gateway Out18/1, Delay/1, AddSub4/3
  Register/1 -> AddSub4/1, delay_val/1, Gateway Out17/1
  Delay/1 -> Register/2
  Gateway Out17/1 -> Scope5/2
  delay_amt/1 -> AddSub4/2, Gateway Out16/1
  Gateway Out16/1 -> Scope5/1, Display1/1
  AddSub4/1 -> Register/1
  Convert3/1 -> Register1/2, Register1/1, Counter/1
  Register1/1 -> Counter/2
  Convert6/1 -> Delay5/1, counter/1, Delay1/1, Delay4/1, Relational2/1, Delay6/1, Delay7/1, Relational5/1

== system exampleModel_bus_axi_w_4ptavg/example/dsp/Cav1/c1p1_PA_conversion ==
  cav_int_q : Inport
  cav_int_i : Inport  Port=2
  ref_int_q : Inport  Port=3
  ref_int_i : Inport  Port=4
  integration_trig : Inport  Port=5
  cal_coefficient : Inport  Port=6
  reset : Inport  Port=7
  AddSub : xbsIndex_r4/AddSub  mode=Subtraction  use_carryin=off  use_carryout=off  en=off  latency=1  precision=User Defined  arith_type="Signed  (2's comp)"  n_bits=18  bin_pt=15  quantization=Truncate  overflow=Wrap  use_behavioral_HDL=off  hw_selection=Fabric  pipelined=off  dbl_ovrd=off  block_type=addsub
  AddSub1 : xbsIndex_r4/AddSub  mode=Addition  use_carryin=off  use_carryout=off  en=off  latency=1  precision=User Defined  arith_type="Signed  (2's comp)"  n_bits=18  bin_pt=15  quantization=Truncate  overflow=Wrap  use_behavioral_HDL=off  hw_selection=Fabric  pipelined=off  dbl_ovrd=off  block_type=addsub
  CORDIC 6.0 1 : xbsIndex_r4/CORDIC 6.0   functional_selection=Translate  architectural_configuration=Parallel  pipelining_mode=Maximum  data_format=SignedFraction  phase_format=Scaled_Radians  input_width=20  output_width=18  round_mode=Truncate  iterations=0  precision=0  compensation_scaling=No_Scale_Compensation  coarse_rotation=on  aclken=off  aresetn=off  out_tready=off  cartesian_has_tuser=off  cartesian_has_tlast=off  cartesian_tuser_width=1  phase_has_tuser=off  phase_has_tlast=off  phase_tuser_width=1  out_tlast_behv=Null  flow_control=NonBlocking  optimize_goal=Resources  trim_axipin_name=on  simulation_type=hybrid_sim  simulation_model=sysgen:cordic_v6_0  data_path_portlist={'s_axis_cartesian_tdata_imag', 's_axis_cartesian_tdata_real', 's_axis_phase_tdata_phase', 'm_axis_dout_tdata_imag', 'm_axis_dout_tdata_real', 'm_axis_dout_tdata_phase','m_axis_dout_tdata'}  ip_name=CORDIC  ip_version=6.0  dsptool_ready=true  ipcore_usecache=true  ipcore_useipmodelcache=true  wrapper_available=true  port_translation_map={ 'aclken' => 'en', 'aresetn' => 'rst' }  block_type=cordic_v6_0
      settings: infoedit=CORDIC 6.0
  CORDIC 6.0 2 : xbsIndex_r4/CORDIC 6.0   functional_selection=Translate  architectural_configuration=Parallel  pipelining_mode=Maximum  data_format=SignedFraction  phase_format=Scaled_Radians  input_width=20  output_width=18  round_mode=Truncate  iterations=0  precision=0  compensation_scaling=No_Scale_Compensation  coarse_rotation=on  aclken=off  aresetn=off  out_tready=off  cartesian_has_tuser=off  cartesian_has_tlast=off  cartesian_tuser_width=1  phase_has_tuser=off  phase_has_tlast=off  phase_tuser_width=1  out_tlast_behv=Null  flow_control=NonBlocking  optimize_goal=Resources  trim_axipin_name=on  simulation_type=hybrid_sim  simulation_model=sysgen:cordic_v6_0  data_path_portlist={'s_axis_cartesian_tdata_imag', 's_axis_cartesian_tdata_real', 's_axis_phase_tdata_phase', 'm_axis_dout_tdata_imag', 'm_axis_dout_tdata_real', 'm_axis_dout_tdata_phase','m_axis_dout_tdata'}  ip_name=CORDIC  ip_version=6.0  dsptool_ready=true  ipcore_usecache=true  ipcore_useipmodelcache=true  wrapper_available=true  port_translation_map={ 'aclken' => 'en', 'aresetn' => 'rst' }  block_type=cordic_v6_0
      settings: infoedit=CORDIC 6.0
  CORDIC 6.0 3 : xbsIndex_r4/CORDIC 6.0   functional_selection=Sin_and_Cos  architectural_configuration=Parallel  pipelining_mode=Maximum  data_format=SignedFraction  phase_format=Scaled_Radians  input_width=18  output_width=18  round_mode=Truncate  iterations=0  precision=0  compensation_scaling=No_Scale_Compensation  coarse_rotation=on  aclken=off  aresetn=off  out_tready=off  cartesian_has_tuser=off  cartesian_has_tlast=off  cartesian_tuser_width=1  phase_has_tuser=off  phase_has_tlast=off  phase_tuser_width=1  out_tlast_behv=Null  flow_control=NonBlocking  optimize_goal=Resources  trim_axipin_name=on  simulation_type=hybrid_sim  simulation_model=sysgen:cordic_v6_0  data_path_portlist={'s_axis_cartesian_tdata_imag', 's_axis_cartesian_tdata_real', 's_axis_phase_tdata_phase', 'm_axis_dout_tdata_imag', 'm_axis_dout_tdata_real', 'm_axis_dout_tdata_phase','m_axis_dout_tdata'}  ip_name=CORDIC  ip_version=6.0  dsptool_ready=true  ipcore_usecache=true  ipcore_useipmodelcache=true  wrapper_available=true  port_translation_map={ 'aclken' => 'en', 'aresetn' => 'rst' }  block_type=cordic_v6_0
      settings: infoedit=CORDIC 6.0
  Constant : xbsIndex_r4/Constant  const=0  gui_display_data_type=Fixed-point  arith_type=Unsigned  n_bits=1  bin_pt=0  preci_type=Single  exp_width=8  frac_width=24  explicit_period=off  period=1  equ=P=C  opselect=C  inp2=PCIN>>17  opr=+  inp1=P  carry=CIN  dbl_ovrd=off  block_type=constant
  Convert : xbsIndex_r4/Convert  gui_display_data_type=Fixed-point  arith_type="Signed  (2's comp)"  n_bits=18  bin_pt=17  float_type=Single  exp_bits=8  fraction_bits=24  quantization=Truncate  overflow=Wrap  en=off  latency=1  pipeline=off  dbl_ovrd=off  block_type=convert
  Convert1 : xbsIndex_r4/Convert  gui_display_data_type=Fixed-point  arith_type="Signed  (2's comp)"  n_bits=18  bin_pt=15  float_type=Single  exp_bits=8  fraction_bits=24  quantization=Truncate  overflow=Wrap  en=off  latency=1  pipeline=off  dbl_ovrd=off  block_type=convert
  Delay{,1..4} (5 alike) : xbsIndex_r4/Delay  rst=off  infoeditControl=Selection of Reset will increase slice count due to use of real FFs and instead of SRLs  en=off  latency=1  reg_retiming=off  dbl_ovrd=off  block_type=delay
  Gateway Out{1..7,10..11} (9 alike) : xbsIndex_r4/Gateway Out  inherit_from_input=off  hdl_port=off  rows=1  columns=1  UseAsDAC=off  DACChannel='1'  interface=None  automatic_assignment=on  address_offset=hex2dec('00')  intf_name=''  intf_description=''  timing_constraint=None  locs_specified=off  LOCs={}  io_standard={}  block_type=gatewayout
  Register{1..5,11} (6 alike) : xbsIndex_r4/Register  init=0  rst=on  en=on  dbl_ovrd=off  block_type=register
  Register6 : xbsIndex_r4/Register  init=0  rst=on  en=off  dbl_ovrd=off  block_type=register
  Relational : xbsIndex_r4/Relational  mode=a!=b  op_type=Bool  en=off  latency=2  dbl_ovrd=off  block_type=relational
  Scope1 : Scope  NumInputPorts=3
  Scope2 : Scope  NumInputPorts=3
  Scope4 : Scope  NumInputPorts=3
  Subsystem : Subsystem
  Subsystem1 : Subsystem
  Subsystem2 : Subsystem
  phi_diff : Outport
  ref_phi_out : Outport  Port=2
  ref_amp_out : Outport  Port=3
  cav_phi_out : Outport  Port=4
  cav_amp_out : Outport  Port=5
  phi_diff_Q : Outport  Port=6
  phi_diff_I : Outport  Port=7
  wires:
  CORDIC 6.0 2/3 -> Delay2/1
  CORDIC 6.0 1/3 -> Delay/1
  CORDIC 6.0 2/2 -> Delay3/1
  Subsystem/1(Out1) -> Gateway Out1/1, Register2/3, Register3/3
  [trig] -> CORDIC 6.0 1/1
  cav_int_q/1 -> CORDIC 6.0 1/2
  ref_int_i/1 -> CORDIC 6.0 2/3
  CORDIC 6.0 1/2 -> Delay1/1
  cav_int_i/1 -> CORDIC 6.0 1/3
  ref_int_q/1 -> CORDIC 6.0 2/2
  Delay/1 -> Register3/1
  Delay1/1 -> Register2/1
  Delay2/1 -> Register1/1
  Delay3/1 -> Register11/1
  [ref_phi_out] -> Delay4/1
  AddSub/1 -> Register6/1, Relational/1, Convert/1, Gateway Out5/1
  [trig] -> CORDIC 6.0 2/1
  integration_trig/1 -> [trig]
  AddSub1/1 -> Gateway Out4/1, AddSub/1
  [cav_phi_out] -> AddSub1/1
  cal_coefficient/1 -> AddSub1/2
  Register11/1 -> [ref_phi_out], ref_phi_out/1
  Register1/1 -> ref_amp_out/1
  Register2/1 -> Gateway Out2/1, [cav_phi_out], cav_phi_out/1
  Register3/1 -> cav_amp_out/1
  CORDIC 6.0 3/3 -> Register5/1
  CORDIC 6.0 3/2 -> Register4/1
  reset/1 -> [B_reset]
  [B_reset] -> Register1/2, Register11/2
  [B_reset] -> Register3/2, Register2/2
  Register4/1 -> Gateway Out10/1, phi_diff_Q/1
  Register5/1 -> Gateway Out11/1, phi_diff_I/1
  Register6/1 -> Gateway Out6/1, phi_diff/1
  [B_reset] -> Register5/2, Register4/2, Register6/2
  CORDIC 6.0 1/1 -> Subsystem/1(In1)
  CORDIC 6.0 2/1 -> Subsystem2/1(In1)
  Delay4/1 -> AddSub/2
  Subsystem2/1(Out1) -> Register1/3, Register11/3
  Convert/1 -> Convert1/1
  Convert1/1 -> CORDIC 6.0 3/2
  Gateway Out10/1 -> Scope4/1
  Gateway Out11/1 -> Scope4/2
  Gateway Out2/1 -> Scope1/2
  Gateway Out1/1 -> Scope1/1
  [B_reset] -> Gateway Out3/1
  Gateway Out3/1 -> Scope1/3
  Gateway Out5/1 -> Scope2/2
  Gateway Out4/1 -> Scope2/1
  Relational/1 -> CORDIC 6.0 3/1
  Gateway Out6/1 -> Scope2/3
  Gateway Out7/1 -> Scope4/3
  Constant/1 -> Relational/2
  CORDIC 6.0 3/1 -> Subsystem1/1(In1)
  Subsystem1/1(Out1) -> Register5/3, Register4/3, Gateway Out7/1

== system exampleModel_bus_axi_w_4ptavg/example/dsp/Cav1/c1p1_freq_err_module ==
  imag : Inport
  real : Inport  Port=2
  flo_window : Inport  Port=3
  reset : Inport  Port=4
  CORDIC 6.0 2 : xbsIndex_r4/CORDIC 6.0   functional_selection=Translate  architectural_configuration=Parallel  pipelining_mode=Maximum  data_format=SignedFraction  phase_format=Scaled_Radians  input_width=18  output_width=18  round_mode=Truncate  iterations=0  precision=0  compensation_scaling=No_Scale_Compensation  coarse_rotation=on  aclken=off  aresetn=off  out_tready=off  cartesian_has_tuser=off  cartesian_has_tlast=off  cartesian_tuser_width=1  phase_has_tuser=off  phase_has_tlast=off  phase_tuser_width=1  out_tlast_behv=Null  flow_control=NonBlocking  optimize_goal=Resources  trim_axipin_name=on  simulation_type=hybrid_sim  simulation_model=sysgen:cordic_v6_0  data_path_portlist={'s_axis_cartesian_tdata_imag', 's_axis_cartesian_tdata_real', 's_axis_phase_tdata_phase', 'm_axis_dout_tdata_imag', 'm_axis_dout_tdata_real', 'm_axis_dout_tdata_phase','m_axis_dout_tdata'}  ip_name=CORDIC  ip_version=6.0  dsptool_ready=true  ipcore_usecache=true  ipcore_useipmodelcache=true  wrapper_available=true  port_translation_map={ 'aclken' => 'en', 'aresetn' => 'rst' }  block_type=cordic_v6_0
      settings: infoedit=CORDIC 6.0
  Clock Enable Probe4 : xbsIndex_r4/Clock Enable Probe  inherit_constraints=on  block_type=ceprobe
      settings: infoedit="Clock enable extractor.  Produces a Boolean output that mirrors the hardware clock enable associated with the input sample rate.<br><br>Hardware notes: in hardware this block costs nothing."
  Down Sample5 : xbsIndex_r4/Down Sample  sample_ratio=12  sample_phase="Last Value of Frame  (most efficient)"  en=off  rst=off  latency=1  dbl_ovrd=off  block_type=dsamp
  Gateway Out{1,38,41,53} (4 alike) : xbsIndex_r4/Gateway Out  inherit_from_input=off  hdl_port=off  rows=1  columns=1  UseAsDAC=off  DACChannel='1'  interface=None  automatic_assignment=on  address_offset=hex2dec('00')  intf_name=''  intf_description=''  timing_constraint=None  locs_specified=off  LOCs={}  io_standard={}  block_type=gatewayout
  Gateway Out44 : xbsIndex_r4/Gateway Out  inherit_from_input=off  hdl_port=on  rows=1  columns=1  UseAsDAC=off  DACChannel='1'  interface=None  automatic_assignment=on  address_offset=hex2dec('00')  intf_name=''  intf_description=''  timing_constraint=None  locs_specified=off  LOCs={}  io_standard={}  block_type=gatewayout
  Gateway Out46 : xbsIndex_r4/Gateway Out  inherit_from_input=off  hdl_port=on  rows=1  columns=1  UseAsDAC=off  DACChannel='1'  interface=None  automatic_assignment=on  address_offset=hex2dec('00')  intf_name=''  intf_description=''  timing_constraint=None  locs_specified=off  LOCs={}  io_standard={}  block_type=gatewayout
  Scope21 : Scope  NumInputPorts=4
  Scope22 : Scope  NumInputPorts=2
  freq_err1 : Subsystem
  NCO_err_fb : Outport
  freq_err : Outport  Port=2
  wires:
  [c1p2_pt_cntr] -> Gateway Out41/1
  Down Sample5/1 -> CORDIC 6.0 2/1
  Gateway Out38/1 -> Scope21/2
  reset/1 -> freq_err1/3(reset)
  CORDIC 6.0 2/3 -> Gateway Out53/1
  Clock Enable Probe4/1 -> Down Sample5/1
  CORDIC 6.0 2/2 -> freq_err1/1(raw_phase), Gateway Out38/1
  real/1 -> CORDIC 6.0 2/3, Gateway Out44/1
  imag/1 -> CORDIC 6.0 2/2, Clock Enable Probe4/1, Gateway Out46/1
  flo_window/1 -> Gateway Out1/1, freq_err1/2(window)
  Gateway Out44/1 -> Scope22/2
  Gateway Out53/1 -> Scope21/1
  Gateway Out41/1 -> Scope21/3
  freq_err1/1(NCO_err) -> NCO_err_fb/1
  Gateway Out46/1 -> Scope22/1
  freq_err1/2(freq_err) -> freq_err/1
  Gateway Out1/1 -> Scope21/4
